simulink model "maglev"  (R2018a)
settings: Solver=VariableStepAuto  StartTime=0.0  StopTime=10.0  RelTol=1e-3
settings Model: Creator=armooga4  LastModifiedBy=armooga4

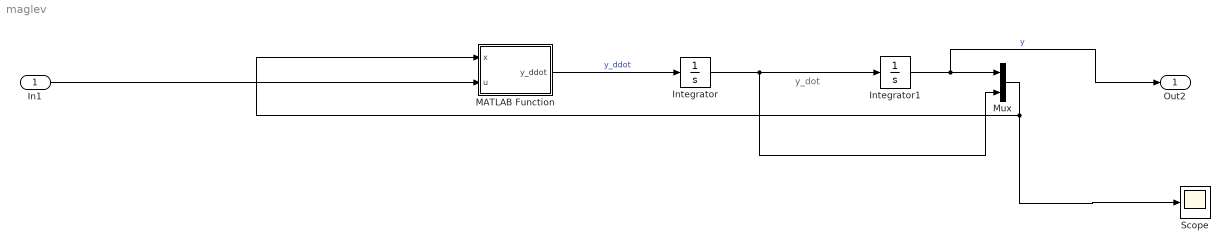
== system maglev ==
  note: y_dot
  In1 : Inport
  Integrator : Integrator  InitialCondition=0.5
  Integrator1 : Integrator  InitialCondition=1.3
  MATLAB Function : MATLAB Function  TreatAsAtomicUnit=on
  Mux : Mux  Inputs=2
  Scope : Scope
  Out2 : Outport  VectorParamsAs1DForOutWhenUnconnected=on
  wires:
  MATLAB Function/1(y_ddot) -> Integrator/1  "y_ddot"
  Mux/1 -> Scope/1, MATLAB Function/1(x)
  Integrator1/1 -> Out2/1, Mux/1  "y"
  In1/1 -> MATLAB Function/2(u)
  Integrator/1 -> Mux/2, Integrator1/1

== matlab function maglev/MATLAB Function ==
  data: x input; u input; y_ddot output
function y_ddot = fcn(x, u)

y_ddot = 9.8 - ((u^2)/(x(1)^2));
